simulink model "simulink_full_observer"  (R2021b)
settings: Solver=VariableStepAuto  StartTime=0.0  StopTime=10  RelTol=1e-3
values from neighbouring files (symbols this model uses):
  A = [0, 0, 0, 1, 0, 0 ... (first row only)    [basic_data.m]    (also in basic_data.mat = [0 0 0 0 -22.4688936865 5 0 0 0 6.5 19.3959496459 -3.6 ... (; lqr.mat = [0 0 0 0 -22.4688936865 5 0 0 0 6.5 19.3959496459 -3.6 ... ()
  B = [0, 0 ... (first row only)    [basic_data.m]    (also in basic_data.mat = [0  0; 0  0; 0  0; 27  11.2; 6.06660129535  -1.63757677119; ; lqr.mat = [0  0; 0  0; 0  0; 27  11.2; 6.06660129535  -1.63757677119; )
  C = [1, 0, 0, 0, 0, 0 ... (first row only)    [basic_data.m]    (also in basic_data.mat = [1 0 0 0 1 0 0 0 1 0 0 0 ... (18 elements, 3x6)]; lqr.mat = [1 0 0 0 1 0 0 0 1 0 0 0 ... (18 elements, 3x6)])
  K = real(inv(R)*B'*P)    [ARE.m]    (also in LQR.m = inv(R)*B'*P; Pole_Placement_function.m = h/Wc*S; decoupled.m = F*C_star_star; lqr.mat = [-254.853126299  165.420589601  161.115517614  -14.472900470)
  L = [-7.81254179223 3.10130437668 1.25751581924 111.669383127 37.0381635845 -11.1796826045 -7.81254179223 3.10130437668 1.25751581924 111.669383127 37.0381635845 -11.1796826045 ... (18 elements, 6x3)]    [L.mat]    (also in observer.m = (v*Pole_Placement(A',C'*v,p))')
  x_0 = [0.2, -0.1, 0.15, -1, 0.8, 0]'    [basic_data.m]    (also in basic_data.mat = [0.2 -0.1 0.15 -1 0.8 0]; lqr.mat = [0.2 -0.1 0.15 -1 0.8 0])
settings Model: Creator=asus  LastModifiedBy=asus

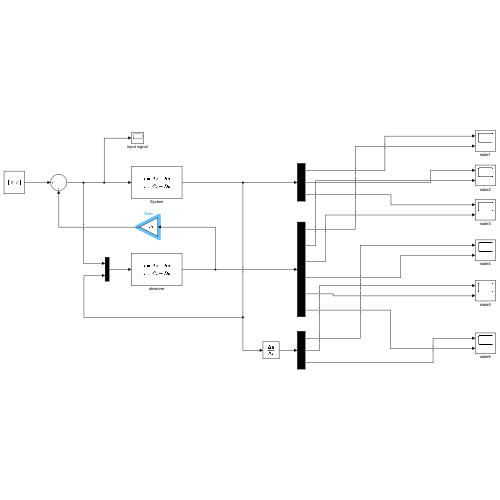
[thumbnail: Simulink's stored preview of the top-level diagram]
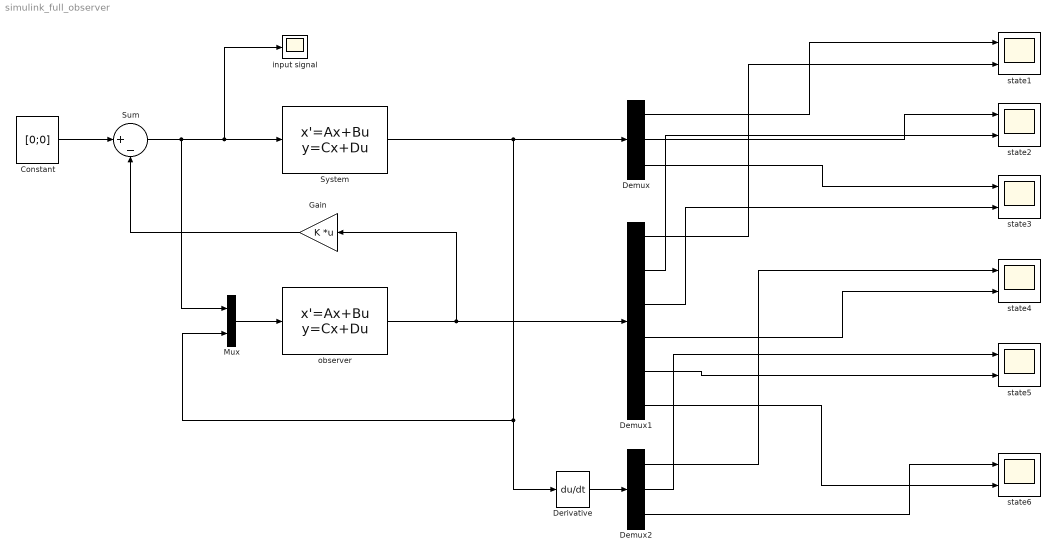
== system simulink_full_observer ==
  Constant : Constant  Value=[0;0]
  Demux : Demux  Outputs=3
  Demux1 : Demux  Outputs=6
  Demux2 : Demux  Outputs=3
  Derivative : Derivative
  Gain : Gain  Gain=K  Multiplication=Matrix(K*u)
  Mux : Mux  Inputs=2
  Sum : Sum  Inputs=|+-
  System : StateSpace  A=A  B=B  C=C  D=zeros(3,2);  InitialCondition=x_0
  input signal : Scope
  observer : StateSpace  A=A-L*C  B=[B L]  C=eye(6)  D=zeros(6,5)  InitialCondition=0
  state{1..6} (6 alike) : Scope  NumInputPorts=2
  wires:
  Sum/1 -> Mux/1, input signal/1, System/1
  Mux/1 -> observer/1
  System/1 -> Derivative/1, Mux/2, Demux/1
  observer/1 -> Demux1/1, Gain/1
  Gain/1 -> Sum/2
  Constant/1 -> Sum/1
  Demux/1 -> state1/1
  Demux/2 -> state2/1
  Demux/3 -> state3/1
  Demux1/1 -> state1/2
  Demux1/2 -> state2/2
  Demux1/3 -> state3/2
  Demux1/4 -> state4/2
  Demux1/5 -> state5/2
  Demux1/6 -> state6/2
  Derivative/1 -> Demux2/1
  Demux2/1 -> state4/1
  Demux2/2 -> state5/1
  Demux2/3 -> state6/1
